simulink model "task2"  (R2024a)
settings: Solver=VariableStepAuto  StartTime=0.0  StopTime=10.0  RelTol=1e-6
values from neighbouring files (symbols this model uses):
  A = [8, 1, 11; 4, 0, 4; -4, -3, -7]    [main.m]
  B = [-1; -3; 3]    [main.m]
  C = [-6, 6, 6, 6; 3, 0, 0, 3]    [main.m]
  K = K4    [main.m]
  L = L2    [main.m]
settings Model: Creator=alexivanov  LastModifiedBy=alexivanov

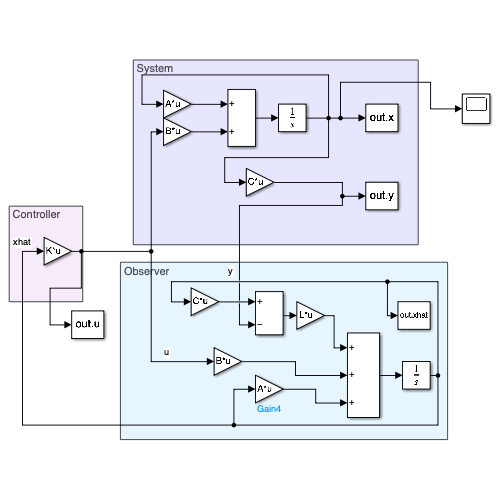
[thumbnail: Simulink's stored preview of the top-level diagram]
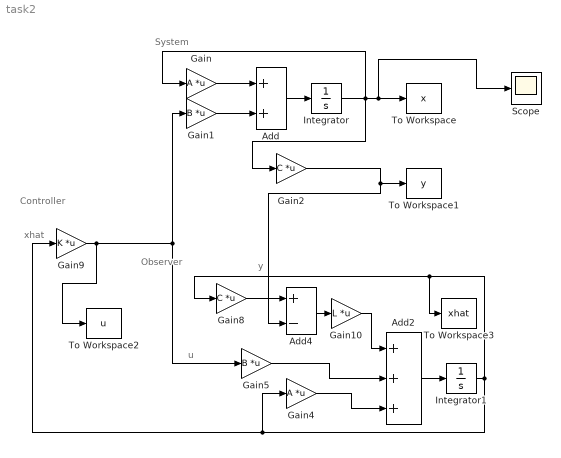
== system task2 ==
  note: Controller
  note: xhat
  note: y
  note: Observer
  note: System
  note: u
  Add : Sum
  Add2 : Sum  Inputs=+++
  Add4 : Sum  Inputs=+-
  Gain : Gain  Gain=A  Multiplication=Matrix(K*u)
  Gain1 : Gain  Gain=B  Multiplication=Matrix(K*u)
  Gain10 : Gain  Gain=L  Multiplication=Matrix(K*u)
  Gain2 : Gain  Gain=C  Multiplication=Matrix(K*u)
  Gain4 : Gain  Gain=A  Multiplication=Matrix(K*u)
  Gain5 : Gain  Gain=B  Multiplication=Matrix(K*u)
  Gain8 : Gain  Gain=C  Multiplication=Matrix(K*u)
  Gain9 : Gain  Gain=K  Multiplication=Matrix(K*u)
  Integrator : Integrator  InitialCondition=[1, 1, 1, 1]
  Integrator1 : Integrator
  Scope : Scope
  To Workspace : ToWorkspace  VariableName=x  SampleTime=-1
  To Workspace1 : ToWorkspace  VariableName=y  SampleTime=-1
  To Workspace2 : ToWorkspace  VariableName=u  SampleTime=-1
  To Workspace3 : ToWorkspace  VariableName=xhat  SampleTime=-1
  wires:
  Gain/1 -> Add/1
  Gain1/1 -> Add/2
  Add/1 -> Integrator/1
  Integrator/1 -> Gain2/1, Scope/1, To Workspace/1, Gain/1
  Gain2/1 -> Add4/2, To Workspace1/1
  Gain9/1 -> Gain1/1, Gain5/1, To Workspace2/1
  Add2/1 -> Integrator1/1
  Integrator1/1 -> Gain9/1, Gain4/1, To Workspace3/1, Gain8/1
  Gain8/1 -> Add4/1
  Gain4/1 -> Add2/3
  Add4/1 -> Gain10/1
  Gain10/1 -> Add2/1
  Gain5/1 -> Add2/2
